simulink model "dp_statefeedback"  (R2015b)
settings: Solver=FixedStepAuto  StartTime=0.0  StopTime=10  FixedStep=T_s  RelTol=1e-3
InitFcn:
  | dp_statefeedback_script
values from neighbouring files (symbols this model uses):
  d_p1 = 0.001    [dp_EKF_script.m]    (also in dp_UKF_script.m; dp_kalman_script.m; dp_real_vs_lin_script.m; dp_statefeedback_script.m)
  d_p2 = 0.001    [dp_EKF_script.m]    (also in dp_UKF_script.m; dp_kalman_script.m; dp_real_vs_lin_script.m; dp_statefeedback_script.m)
  g = 9.81    [dp_EKF_script.m]    (also in dp_UKF_script.m; dp_kalman_script.m; dp_real_vs_lin_script.m; dp_statefeedback_script.m)
  K6 = place(A6,B6,p_s6)    [dp_kalman_script.m]    (also in dp_real_vs_lin_script.m; dp_statefeedback_script.m)
  l_1 = 0.194    [dp_EKF_script.m]    (also in dp_UKF_script.m; dp_kalman_script.m; dp_real_vs_lin_script.m; dp_statefeedback_script.m)
  l_2 = 0.1855    [dp_EKF_script.m]    (also in dp_UKF_script.m; dp_kalman_script.m; dp_real_vs_lin_script.m; dp_statefeedback_script.m)
  m_1 = 0.0313    [dp_EKF_script.m]    (also in dp_UKF_script.m; dp_kalman_script.m; dp_real_vs_lin_script.m; dp_statefeedback_script.m)
  m_2 = 0.0313    [dp_EKF_script.m]    (also in dp_UKF_script.m; dp_kalman_script.m; dp_real_vs_lin_script.m; dp_statefeedback_script.m)
  m_3 = 0.0308    [dp_EKF_script.m]    (also in dp_UKF_script.m; dp_kalman_script.m; dp_real_vs_lin_script.m; dp_statefeedback_script.m)
  T_s = 0.001    [dp_EKF_script.m]    (also in dp_UKF_script.m; dp_kalman_script.m; dp_real_vs_lin_script.m; dp_statefeedback_script.m)
undefined symbols (not defined in the file or in its folder): DiscIntNeverNeededParam, K6_lqr
settings Model: Creator=serov  LastModifiedBy=serov

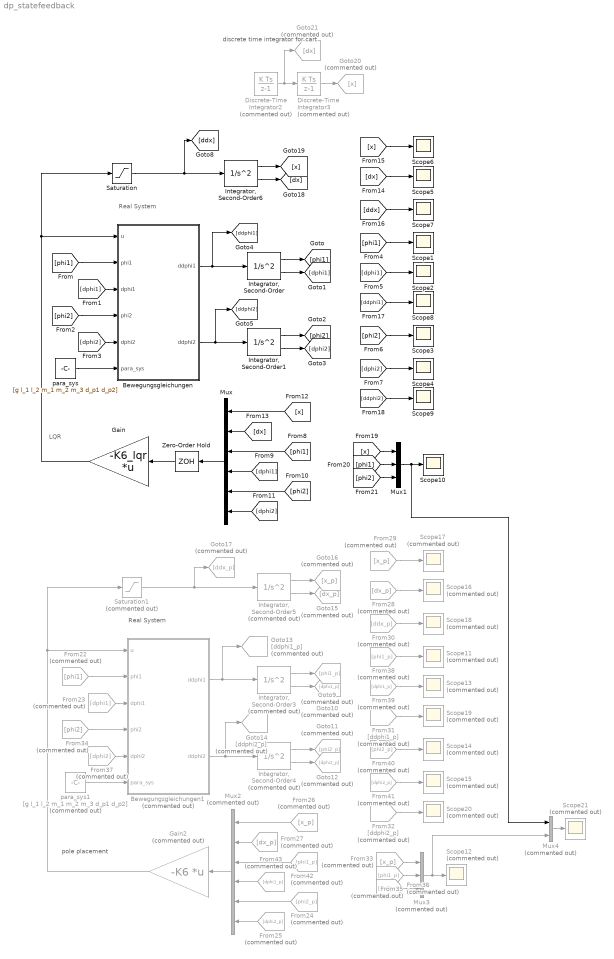
== system dp_statefeedback ==
  note: discrete time integrator for cart
  note: LQR
  note: Real System
  note: pole placement
  note: Real System
  Bewegungsgleichungen : MATLAB Function  TreatAsAtomicUnit=on
  Bewegungsgleichungen1 : MATLAB Function  Commented=on  TreatAsAtomicUnit=on
  Discrete-Time Integrator2 : DiscreteIntegrator  Commented=on  InitialConditionSetting=State (most efficient)  SampleTime=T_s  LimitOutput=on  UpperSaturationLimit=5  LowerSaturationLimit=-5  ICPrevOutput=DiscIntNeverNeededParam  ICPrevScaledInput=DiscIntNeverNeededParam
  Discrete-Time Integrator3 : DiscreteIntegrator  Commented=on  InitialConditionSetting=State (most efficient)  SampleTime=T_s  LimitOutput=on  UpperSaturationLimit=0.2  LowerSaturationLimit=-0.2  ICPrevOutput=DiscIntNeverNeededParam  ICPrevScaledInput=DiscIntNeverNeededParam
  From22 : From  Commented=on  GotoTag=phi1
  From23 : From  Commented=on  GotoTag=dphi1
  From24 : From  Commented=on  GotoTag=phi2_p
  From25 : From  Commented=on  GotoTag=dphi2_p
  From26 : From  Commented=on  GotoTag=x_p
  From27 : From  Commented=on  GotoTag=dx_p
  From28 : From  Commented=on  GotoTag=dx_p
  From29 : From  Commented=on  GotoTag=x_p
  From30 : From  Commented=on  GotoTag=ddx_p
  From31 : From  Commented=on  GotoTag=ddphi1_p
  From32 : From  Commented=on  GotoTag=ddphi2_p
  From33 : From  Commented=on  GotoTag=x_p
  From34 : From  Commented=on  GotoTag=phi2
  From35 : From  Commented=on  GotoTag=phi1_p
  From36 : From  Commented=on  GotoTag=phi2_p
  From37 : From  Commented=on  GotoTag=dphi2
  From38 : From  Commented=on  GotoTag=phi1_p
  From39 : From  Commented=on  GotoTag=dphi1_p
  From40 : From  Commented=on  GotoTag=phi2_p
  From41 : From  Commented=on  GotoTag=dphi2_p
  From42 : From  Commented=on  GotoTag=phi1_p
  From43 : From  Commented=on  GotoTag=dphi1_p
  Gain : Gain  Gain=-K6_lqr  Multiplication=Matrix(K*u) (u vector)
  Gain2 : Gain  Commented=on  Gain=-K6  Multiplication=Matrix(K*u) (u vector)
  Goto10 : Goto  Commented=on  GotoTag=dphi1_p
  Goto11 : Goto  Commented=on  GotoTag=phi2_p
  Goto12 : Goto  Commented=on  GotoTag=dphi2_p
  Goto13 : Goto  Commented=on  GotoTag=ddphi1_p
  Goto14 : Goto  Commented=on  GotoTag=ddphi2_p
  Goto15 : Goto  Commented=on  GotoTag=dx_p
  Goto16 : Goto  Commented=on  GotoTag=x_p
  Goto17 : Goto  Commented=on  GotoTag=ddx_p
  Goto20 : Goto  Commented=on  GotoTag=x
  Goto21 : Goto  Commented=on  GotoTag=dx
  Goto9 : Goto  Commented=on  GotoTag=phi1_p
  "Integrator, Second-Order" : SecondOrderIntegrator  ICX=phi1_0  ICDXDT=dphi1_0
  "Integrator, Second-Order1" : SecondOrderIntegrator  ICX=phi2_0  ICDXDT=dphi2_0
  "Integrator, Second-Order3" : SecondOrderIntegrator  Commented=on  ICX=phi1_0  ICDXDT=dphi1_0
  "Integrator, Second-Order4" : SecondOrderIntegrator  Commented=on  ICX=phi2_0  ICDXDT=dphi2_0
  "Integrator, Second-Order5" : SecondOrderIntegrator  Commented=on  ICX=x_0  LimitX=on  UpperLimitX=0.2  LowerLimitX=-0.2  ICDXDT=dx_0  LimitDXDT=on  UpperLimitDXDT=5  LowerLimitDXDT=-5
  "Integrator, Second-Order6" : SecondOrderIntegrator  ICX=x_0  LimitX=on  UpperLimitX=0.2  LowerLimitX=-0.2  ICDXDT=dx_0  LimitDXDT=on  UpperLimitDXDT=5  LowerLimitDXDT=-5
  Mux : Mux  Inputs=6
  Mux1 : Mux  Inputs=3
  Mux2 : Mux  Commented=on  Inputs=6
  Mux3 : Mux  Commented=on  Inputs=3
  Mux4 : Mux  Commented=on  Inputs=2
  Saturation : Saturate  UpperLimit=20  LowerLimit=-20
  Saturation1 : Saturate  Commented=on  UpperLimit=20  LowerLimit=-20
  Scope{1..10} (10 alike) : Scope
  Scope{11..21} (11 alike) : Scope  Commented=on
  Zero-Order Hold : ZeroOrderHold  SampleTime=T_s
  para_sys : Constant  Value=[g l_1 l_2 m_1 m_2 m_3 d_p1 d_p2]
  para_sys1 : Constant  Commented=on  Value=[g l_1 l_2 m_1 m_2 m_3 d_p1 d_p2]
  wires:
  Bewegungsgleichungen/1(ddphi1) -> [ddphi1], "Integrator, Second-Order"/1
  Bewegungsgleichungen/2(ddphi2) -> [ddphi2], "Integrator, Second-Order1"/1
  "Integrator, Second-Order"/1 -> [phi1]
  "Integrator, Second-Order"/2 -> [dphi1]
  "Integrator, Second-Order1"/2 -> [dphi2]
  "Integrator, Second-Order1"/1 -> [phi2]
  [phi1] -> Bewegungsgleichungen/2(phi1)
  [dphi1] -> Bewegungsgleichungen/3(dphi1)
  [phi2] -> Bewegungsgleichungen/4(phi2)
  [dphi2] -> Bewegungsgleichungen/5(dphi2)
  para_sys/1 -> Bewegungsgleichungen/6(para_sys)
  [phi1] -> Scope1/1
  [dphi1] -> Scope2/1
  [phi2] -> Scope3/1
  [dphi2] -> Scope4/1
  [phi1] -> Mux/3
  [dphi1] -> Mux/4
  [phi2] -> Mux/5
  [dphi2] -> Mux/6
  Mux/1 -> Zero-Order Hold/1
  [x] -> Mux/1
  [dx] -> Mux/2
  Gain/1 -> Saturation/1, Bewegungsgleichungen/1(u)
  [dx] -> Scope5/1
  [x] -> Scope6/1
  [ddx] -> Scope7/1
  [ddphi1] -> Scope8/1
  [ddphi2] -> Scope9/1
  Saturation/1 -> "Integrator, Second-Order6"/1, [ddx]
  Mux1/1 -> Mux4/1, Scope10/1
  [x] -> Mux1/1
  [phi1] -> Mux1/2
  [phi2] -> Mux1/3
  Bewegungsgleichungen1/1(ddphi1) -> Goto13/1, "Integrator, Second-Order3"/1
  Bewegungsgleichungen1/2(ddphi2) -> Goto14/1, "Integrator, Second-Order4"/1
  "Integrator, Second-Order3"/1 -> Goto9/1
  "Integrator, Second-Order3"/2 -> Goto10/1
  "Integrator, Second-Order4"/2 -> Goto12/1
  "Integrator, Second-Order4"/1 -> Goto11/1
  From22/1 -> Bewegungsgleichungen1/2(phi1)
  From23/1 -> Bewegungsgleichungen1/3(dphi1)
  From34/1 -> Bewegungsgleichungen1/4(phi2)
  From37/1 -> Bewegungsgleichungen1/5(dphi2)
  para_sys1/1 -> Bewegungsgleichungen1/6(para_sys)
  From38/1 -> Scope11/1
  From39/1 -> Scope13/1
  From40/1 -> Scope14/1
  From41/1 -> Scope15/1
  From42/1 -> Mux2/3
  From43/1 -> Mux2/4
  From24/1 -> Mux2/5
  From25/1 -> Mux2/6
  "Integrator, Second-Order5"/1 -> Goto16/1
  "Integrator, Second-Order5"/2 -> Goto15/1
  From26/1 -> Mux2/1
  From27/1 -> Mux2/2
  Mux2/1 -> Gain2/1
  From28/1 -> Scope16/1
  From29/1 -> Scope17/1
  From30/1 -> Scope18/1
  From31/1 -> Scope19/1
  From32/1 -> Scope20/1
  Saturation1/1 -> Goto17/1, "Integrator, Second-Order5"/1
  Mux3/1 -> Mux4/2, Scope12/1
  From33/1 -> Mux3/1
  From35/1 -> Mux3/2
  From36/1 -> Mux3/3
  Gain2/1 -> Saturation1/1, Bewegungsgleichungen1/1(u)
  Mux4/1 -> Scope21/1
  Zero-Order Hold/1 -> Gain/1
  "Integrator, Second-Order6"/1 -> [x]
  "Integrator, Second-Order6"/2 -> [dx]
  ? -> Discrete-Time Integrator2/1
  Discrete-Time Integrator2/1 -> Discrete-Time Integrator3/1, Goto21/1
  Discrete-Time Integrator3/1 -> Goto20/1

== matlab function dp_statefeedback/Bewegungsgleichungen1 ==
  data: u input; phi1 input; dphi1 input; phi2 input; dphi2 input; para_sys input; ddphi1 output; ddphi2 output
function [ddphi1, ddphi2] = pendel_1_2(u, phi1, dphi1, phi2, dphi2, para_sys)
%#codegen

g = para_sys(1);
l_1 = para_sys(2);
l_2 = para_sys(3);
m_1 = para_sys(4);
m_2 = para_sys(5);
m_3 = para_sys(6);
d_p1 = para_sys(7);
d_p2 = para_sys(8);

ddphi1 = 1/(l_1^2*(9*cos(phi1-phi2)^2*m_2-4*m_1-12*m_2-12*m_3)*l_2)*(9*dphi1^2*cos(phi1-phi2)*sin(phi1-phi2)*l_1^2*l_2*m_2+6*m_2*l_1*l_2^2*sin(phi1-phi2)*dphi2^2+9*u*cos(phi1-phi2)*cos(phi2)*l_1*l_2*m_2+9*cos(phi1-phi2)*sin(phi2)*g*l_1*l_2*m_2-6*l_1*cos(phi1)*u*m_1*l_2-12*l_1*cos(phi1)*u*m_2*l_2-12*l_1*cos(phi1)*u*m_3*l_2-6*l_1*g*sin(phi1)*m_1*l_2-12*l_1*g*sin(phi1)*m_2*l_2-12*l_1*g*sin(phi1)*m_3*l_2+18*dphi1*cos(phi1-phi2)*d_p2*l_1-18*dphi2*cos(phi1-phi2)*d_p2*l_1+12*dphi1*d_p1*l_2+12*dphi1*d_p2*l_2-12*d_p2*dphi2*l_2);

ddphi2 = -1/(l_1*l_2^2*(9*cos(phi1-phi2)^2*m_2-4*m_1-12*m_2-12*m_3)*m_2)*(12*dphi1*d_p2*l_1*m_1+36*dphi1*d_p2*l_1*m_2+36*dphi1*d_p2*l_1*m_3-12*dphi2*d_p2*l_1*m_1-36*dphi2*d_p2*l_1*m_2-36*dphi2*d_p2*l_1*m_3-9*cos(phi1)*u*cos(phi1-phi2)*l_1*l_2*m_1*m_2-18*cos(phi1)*u*cos(phi1-phi2)*l_1*l_2*m_2*m_3-9*cos(phi1-phi2)*sin(phi1)*g*l_1*l_2*m_1*m_2-18*cos(phi1-phi2)*sin(phi1)*g*l_1*l_2*m_2*m_3+9*dphi2^2*cos(phi1-phi2)*sin(phi1-phi2)*l_1*l_2^2*m_2^2+ 6*dphi1^2*sin(phi1-phi2)*l_1^2*l_2*m_1*m_2+ 18*dphi1^2*sin(phi1-phi2)*l_1^2*l_2*m_2*m_3-18*cos(phi1)*u*cos(phi1-phi2)*l_1*l_2*m_2^2-18*cos(phi1-phi2)*sin(phi1)*g*l_1*l_2*m_2^2 +6*u*cos(phi2)*l_1*l_2*m_1*m_2+18*u*cos(phi2)*l_1*l_2*m_2*m_3+6*sin(phi2)*g*l_1*l_2*m_1*m_2+18*sin(phi2)*g*l_1*l_2*m_2*m_3 + 18*(dphi1)^2*sin(phi1-phi2)*l_1^2*l_2*m_2^2+18*u*cos(phi2)*l_1*l_2*m_2^2+18*sin(phi2)*g*l_1*l_2*m_2^2+18*dphi1*cos(phi1-phi2)*d_p1*l_2*m_2 + 18*dphi1*cos(phi1-phi2)*d_p2*l_2*m_2-18*dphi2*cos(phi1-phi2)*d_p2*l_2*m_2);

== matlab function dp_statefeedback/Bewegungsgleichungen ==
  data: u input; phi1 input; dphi1 input; phi2 input; dphi2 input; para_sys input; ddphi1 output; ddphi2 output
function [ddphi1, ddphi2] = pendel_1_2(u, phi1, dphi1, phi2, dphi2, para_sys)
%#codegen

g = para_sys(1);
l_1 = para_sys(2);
l_2 = para_sys(3);
m_1 = para_sys(4);
m_2 = para_sys(5);
m_3 = para_sys(6);
d_p1 = para_sys(7);
d_p2 = para_sys(8);

ddphi1 = 1/(l_1^2*(9*cos(phi1-phi2)^2*m_2-4*m_1-12*m_2-12*m_3)*l_2)*(9*dphi1^2*cos(phi1-phi2)*sin(phi1-phi2)*l_1^2*l_2*m_2+6*m_2*l_1*l_2^2*sin(phi1-phi2)*dphi2^2+9*u*cos(phi1-phi2)*cos(phi2)*l_1*l_2*m_2+9*cos(phi1-phi2)*sin(phi2)*g*l_1*l_2*m_2-6*l_1*cos(phi1)*u*m_1*l_2-12*l_1*cos(phi1)*u*m_2*l_2-12*l_1*cos(phi1)*u*m_3*l_2-6*l_1*g*sin(phi1)*m_1*l_2-12*l_1*g*sin(phi1)*m_2*l_2-12*l_1*g*sin(phi1)*m_3*l_2+18*dphi1*cos(phi1-phi2)*d_p2*l_1-18*dphi2*cos(phi1-phi2)*d_p2*l_1+12*dphi1*d_p1*l_2+12*dphi1*d_p2*l_2-12*d_p2*dphi2*l_2);

ddphi2 = -1/(l_1*l_2^2*(9*cos(phi1-phi2)^2*m_2-4*m_1-12*m_2-12*m_3)*m_2)*(12*dphi1*d_p2*l_1*m_1+36*dphi1*d_p2*l_1*m_2+36*dphi1*d_p2*l_1*m_3-12*dphi2*d_p2*l_1*m_1-36*dphi2*d_p2*l_1*m_2-36*dphi2*d_p2*l_1*m_3-9*cos(phi1)*u*cos(phi1-phi2)*l_1*l_2*m_1*m_2-18*cos(phi1)*u*cos(phi1-phi2)*l_1*l_2*m_2*m_3-9*cos(phi1-phi2)*sin(phi1)*g*l_1*l_2*m_1*m_2-18*cos(phi1-phi2)*sin(phi1)*g*l_1*l_2*m_2*m_3+9*dphi2^2*cos(phi1-phi2)*sin(phi1-phi2)*l_1*l_2^2*m_2^2+ 6*dphi1^2*sin(phi1-phi2)*l_1^2*l_2*m_1*m_2+ 18*dphi1^2*sin(phi1-phi2)*l_1^2*l_2*m_2*m_3-18*cos(phi1)*u*cos(phi1-phi2)*l_1*l_2*m_2^2-18*cos(phi1-phi2)*sin(phi1)*g*l_1*l_2*m_2^2 +6*u*cos(phi2)*l_1*l_2*m_1*m_2+18*u*cos(phi2)*l_1*l_2*m_2*m_3+6*sin(phi2)*g*l_1*l_2*m_1*m_2+18*sin(phi2)*g*l_1*l_2*m_2*m_3 + 18*(dphi1)^2*sin(phi1-phi2)*l_1^2*l_2*m_2^2+18*u*cos(phi2)*l_1*l_2*m_2^2+18*sin(phi2)*g*l_1*l_2*m_2^2+18*dphi1*cos(phi1-phi2)*d_p1*l_2*m_2 + 18*dphi1*cos(phi1-phi2)*d_p2*l_2*m_2-18*dphi2*cos(phi1-phi2)*d_p2*l_2*m_2);
